simulink model "MPC_control"  (R2024b)
settings: Solver=VariableStepAuto  StartTime=0.0  StopTime=15  RelTol=1e-3
libraries: Solver_SF x1
settings Model: Creator=13349  LastModifiedBy=13706
settings SolverCC: AlgebraicLoopSolver=TrustRegion
settings DebuggingCC: ArithmeticOperatorsInVariantConditions=warning
settings ModelReferenceCC: EnableRefExpFcnMdlSchedulingChecks=on
settings SFSimCC: CustomCodeUndefinedFunction=UseInterfaceOnly
settings RTWCC: GPUComputeCapability=3.5

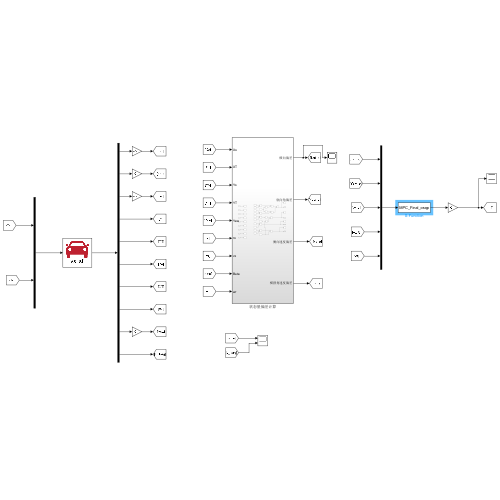
[thumbnail: Simulink's stored preview of the top-level diagram]
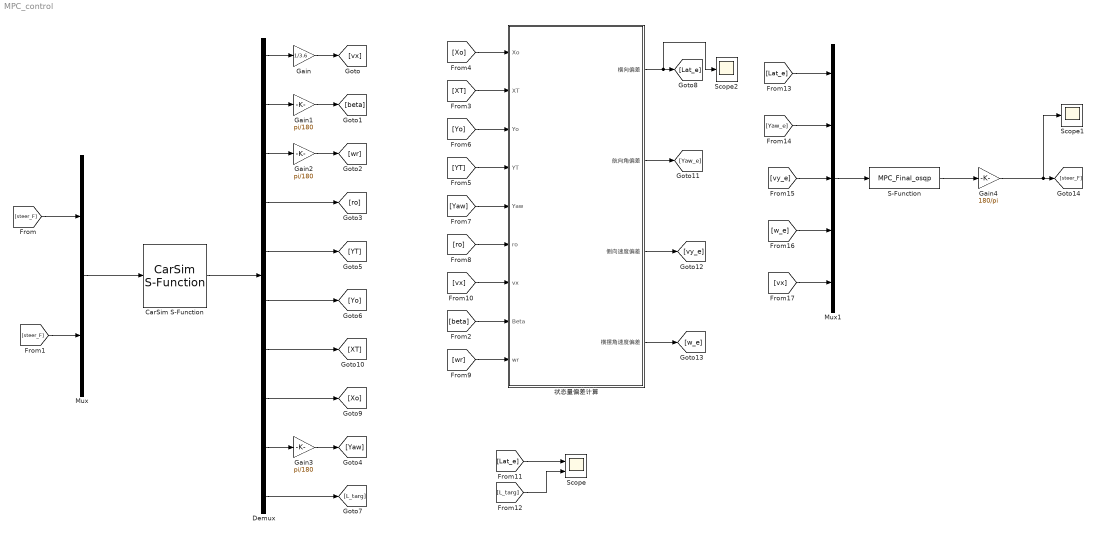
== system MPC_control ==
  CarSim S-Function : Solver_SF/CarSim S-Function  Priority=1  SIMFILE=simfile.sim  Run_RTs=off  vs_state_ind=Run  StopMode_ind=Vehicle Model
  Demux : Demux  Outputs=10
  Gain : Gain  Gain=1/3.6
  Gain1 : Gain  Gain=pi/180
  Gain2 : Gain  Gain=pi/180
  Gain3 : Gain  Gain=pi/180
  Gain4 : Gain  Gain=180/pi
  Mux : Mux  Inputs=2
  Mux1 : Mux  Inputs=5
  S-Function : S-Function  FunctionName=MPC_Final_osqp  SFunctionDeploymentMode=off  EnableBusSupport=off
  Scope : Scope  NumInputPorts=2
  Scope1 : Scope
  Scope2 : Scope
  状态量偏差计算 : Subsystem
  wires:
  Mux1/1 -> S-Function/1
  Mux/1 -> CarSim S-Function/1
  Demux/9 -> Gain3/1
  Gain1/1 -> [beta]
  Demux/10 -> [L_targ]
  Gain3/1 -> [Yaw]
  状态量偏差计算/2(航向角偏差) -> [Yaw_e]
  [L_targ] -> Scope/2
  状态量偏差计算/4(横摆角速度偏差) -> [w_e]
  Demux/7 -> [XT]
  [XT] -> 状态量偏差计算/2(XT)
  [Yaw] -> 状态量偏差计算/5(Yaw)
  [YT] -> 状态量偏差计算/4(YT)
  [ro] -> 状态量偏差计算/6(ro)
  Demux/6 -> [Yo]
  [beta] -> 状态量偏差计算/8(Beta)
  [Lat_e] -> Scope/1
  [wr] -> 状态量偏差计算/9(wr)
  Gain/1 -> [vx]
  Demux/5 -> [YT]
  状态量偏差计算/3(侧向速度偏差) -> [vy_e]
  [vx] -> 状态量偏差计算/7(vx)
  状态量偏差计算/1(横向偏差) -> Scope2/1, [Lat_e]
  [Xo] -> 状态量偏差计算/1(Xo)
  Gain2/1 -> [wr]
  [Yo] -> 状态量偏差计算/3(Yo)
  Demux/2 -> Gain1/1
  CarSim S-Function/1 -> Demux/1
  Demux/1 -> Gain/1
  Demux/8 -> [Xo]
  Demux/3 -> Gain2/1
  Demux/4 -> [ro]
  [Lat_e] -> Mux1/1
  [Yaw_e] -> Mux1/2
  [vy_e] -> Mux1/3
  [w_e] -> Mux1/4
  [vx] -> Mux1/5
  S-Function/1 -> Gain4/1
  Gain4/1 -> Scope1/1, [steer_F]
  [steer_F] -> Mux/1
  [steer_F] -> Mux/2

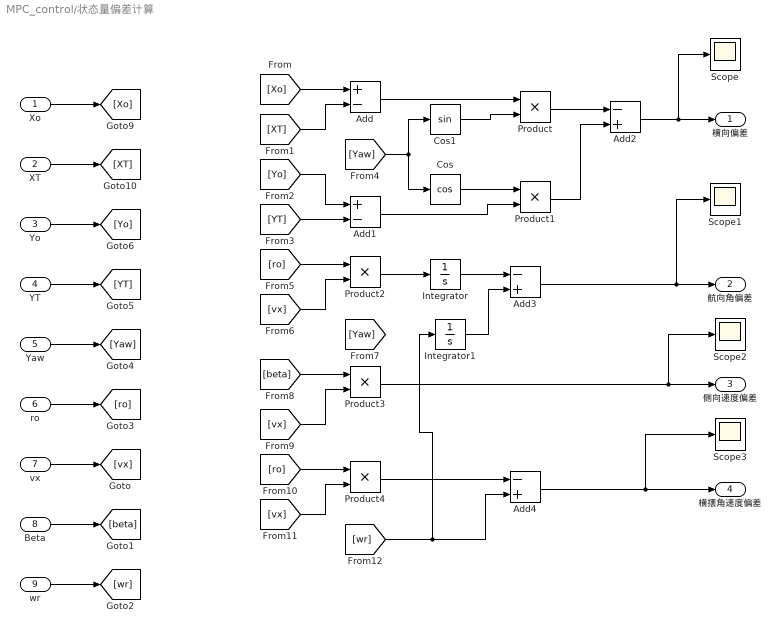
== system MPC_control/状态量偏差计算 ==
  Xo : Inport
  XT : Inport  Port=2
  Yo : Inport  Port=3
  YT : Inport  Port=4
  Yaw : Inport  Port=5
  ro : Inport  Port=6
  vx : Inport  Port=7
  Beta : Inport  Port=8
  wr : Inport  Port=9
  Add : Sum  Inputs=+-
  Add1 : Sum  Inputs=+-
  Add2 : Sum  Inputs=-+
  Add3 : Sum  Inputs=-+
  Add4 : Sum  Inputs=-+
  Cos : Trigonometry  Operator=cos
  Cos1 : Trigonometry
  Integrator : Integrator
  Integrator1 : Integrator
  Product{,1..4} (5 alike) : Product
  Scope{,1..3} (4 alike) : Scope
  横向偏差 : Outport
  航向角偏差 : Outport  Port=2
  侧向速度偏差 : Outport  Port=3
  横摆角速度偏差 : Outport  Port=4
  wires:
  Yaw/1 -> [Yaw]
  Beta/1 -> [beta]
  Xo/1 -> [Xo]
  Yo/1 -> [Yo]
  vx/1 -> [vx]
  ro/1 -> [ro]
  wr/1 -> [wr]
  XT/1 -> [XT]
  YT/1 -> [YT]
  [Xo] -> Add/1
  [XT] -> Add/2
  [Yo] -> Add1/1
  [YT] -> Add1/2
  Add/1 -> Product/1
  Cos1/1 -> Product/2
  [Yaw] -> Cos/1, Cos1/1
  Add1/1 -> Product1/2
  Cos/1 -> Product1/1
  Product/1 -> Add2/1
  Product1/1 -> Add2/2
  Add2/1 -> Scope/1, 横向偏差/1
  [ro] -> Product2/1
  [vx] -> Product2/2
  Product2/1 -> Integrator/1
  Integrator/1 -> Add3/1
  Add3/1 -> Scope1/1, 航向角偏差/1
  [beta] -> Product3/1
  [vx] -> Product3/2
  Product3/1 -> Scope2/1, 侧向速度偏差/1
  Add4/1 -> Scope3/1, 横摆角速度偏差/1
  [wr] -> Integrator1/1, Add4/2
  Product4/1 -> Add4/1
  [vx] -> Product4/2
  [ro] -> Product4/1
  Integrator1/1 -> Add3/2
